simulink model "PI_Controller"  (R2020a)
settings: Solver=VariableStepAuto  StartTime=0.0  StopTime=120  RelTol=1e-3
undefined symbols (not defined in the file or in its folder): Ki, Kp
settings Model: DataDictionary=model_data.sldd  Creator=Viraj  LastModifiedBy=Viraj
settings DataIOCC: SaveOutput=off  SaveTime=off

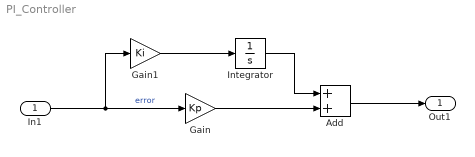
== system PI_Controller ==
  In1 : Inport  OutDataTypeStr=double  PortDimensions=1  SampleTime=0
  Add : Sum
  Gain : Gain  Gain=Kp
  Gain1 : Gain  Gain=Ki
  Integrator : Integrator
  Out1 : Outport  OutDataTypeStr=double  PortDimensions=1  SampleTime=0
  wires:
  In1/1 -> Gain/1, Gain1/1  "error"
  Gain1/1 -> Integrator/1
  Add/1 -> Out1/1
  Gain/1 -> Add/2
  Integrator/1 -> Add/1
